simulink model "m2asm_2_rust"  (R2020b)
settings: Solver=FixedStepDiscrete  StartTime=0.0  StopTime=5  FixedStep=deltaT  RelTol=1e-3
values from neighbouring files (symbols this model uses):
  Cpi_d = c2d(st.asm.fpi,Ts,c2d_opts)    [load_m2asm_data.m]
  fc = 2    [load_m2asm_data.m]
  flag_d = c2d(flag,Ts,c2d_opts)    [load_m2asm_data.m]
  Hpd_d = c2d(st.asm.fpd,Ts,c2d_opts)    [load_m2asm_data.m]
  k2p_stiff = k2p_stiff0    (= 122000000)    [load_m2asm_data.m]
  Km2pS1_dec = Km2p_dec(1:6,1:6)    [load_m2asm_data.m]
  m2p_Cfb_d = c2d(tf(fbH), Ts, 'foh')    [load_m2asm_data.m]
  st = getcontrol_asm()    [load_m2asm_data.m]
  to_diff_m2p_F = kron(eye(6),[1;-1])    [load_m2asm_data.m]
settings Model: SimulationMode=accelerator  Creator=RRomano  LastModifiedBy=rromano
settings DataIOCC: SaveOutput=off  SignalLogging=off  DSMLogging=off  SaveTime=off  ReturnWorkspaceOutputs=off
settings OptimizationCC: StrengthReduction=on  PassReuseOutputArgsAs=Individual arguments  EfficientMapNaN2IntZero=off  SimCompilerOptimization=on  AccelVerboseBuild=on  OptimizeBlockOrder=speed  OptimizationPriority=Speed  OptimizationCustomize=off  MultiThreadedLoops=on  EfficientTunableParamExpr=on
settings DebuggingCC: InheritedTsInSrcMsg=none  MultiTaskRateTransMsg=warning  ParameterTunabilityLossMsg=error  SFUnexpectedBacktrackingDiag=warning  SFNoUnconditionalDefaultTransitionDiag=warning  SFExecutionAtInitializationDiag=none  ArithmeticOperatorsInVariantConditions=warning
settings HardwareCC: ProdBitPerLong=64  ProdHWDeviceType=Intel->x86-64 (Linux 64)  TargetBitPerLong=64  TargetBitPerPointer=64  TargetBitPerSizeT=64  TargetBitPerPtrDiffT=64  TargetLongLongMode=on  TargetIntDivRoundTo=Zero  TargetEndianess=LittleEndian  TargetWordSize=64  TargetHWDeviceType=MATLAB Host  ProdEqTarget=off
settings SFSimCC: SimUseLocalCustomCode=off  MATLABDynamicMemAlloc=off  CustomCodeUndefinedFunction=UseInterfaceOnly
settings RTWCC: Description=Embedded Coder  SystemTargetFile=ert.tlc  GenCodeOnly=on  TemplateMakefile=ert_default_tmf  GenerateReport=on  BuildConfiguration=Faster Runs  IncludeHyperlinkInReport=on  GenerateTraceInfo=on  GenerateTraceReport=on  GenerateTraceReportSl=on  GenerateTraceReportSf=on  GenerateTraceReportEml=on
settings CodeAppCC: ForceParamTrailComments=on  IgnoreCustomStorageClasses=off  MaxIdLength=128  OperatorAnnotations=on  SimulinkDataObjDesc=on  SFDataObjDesc=on  InsertBlockDesc=on  MATLABSourceComments=on
settings ERTTargetCC: GenerateSampleERTMain=on  SuppressErrorStatus=on  CodeInterfacePackaging=Reusable function  RootIOFormat=Structure reference  ERTCustomFileTemplate=example_file_process.tlc
settings ConfigComp: CovMetricSettings=dw  CovSaveCumulativeToWorkspaceVar=on  CovSaveSingleToWorkspaceVar=on  CovExternalEMLEnable=off

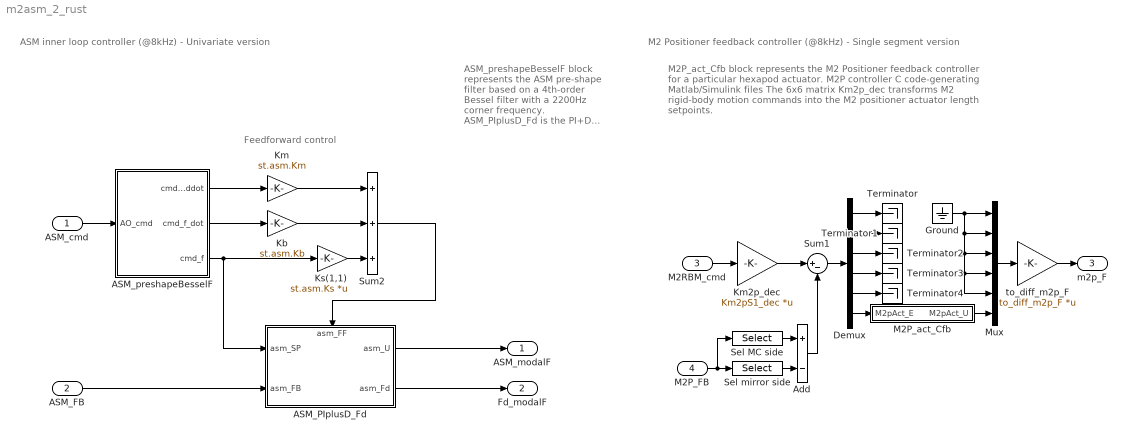
== system m2asm_2_rust ==
  note: Feedforward control
  note: ASM_preshapeBesselF block represents the ASM pre-shape filter based on a 4th-order Bessel filter with a 2200Hz corner frequency.
      | ASM_PIplusD_Fd is the PI+D feedback controller. The block also provides the fluid damping contribution as output asm_Fd .
      | In the modal control approach, Ks is the inverse of the modal stiffness matrix, a square matrix of dimension n_m. Therefore, in that case, Ks(1,1) is just a placeholder.
  note: ASM inner loop controller (@8kHz) - Univariate version
  note: M2 Positioner feedback controller (@8kHz) - Single segment version
  note: M2P_act_Cfb block represents the M2 Positioner feedback controller for a particular hexapod actuator.
      | M2P controller C code-generating Matlab/Simulink files
      | The 6x6 matrix Km2p_dec transforms M2 rigid-body motion commands into the M2 positioner actuator length setpoints.
  ASM_cmd : Inport  Interpolate=off
  ASM_FB : Inport  Port=2
  M2RBM_cmd : Inport  Port=3  Interpolate=off
  M2P_FB : Inport  Port=4
  ASM_PIplusD_Fd : Subsystem
      settings: PortSchema="{\"entries\":[{\"content\":{\"sides\":[{\"content\":{\"connectorIds\":[\"In1\",\"In2\"]},\"type\":\"ConnectorPlacement.EquallySpacedRectSide\",\"uuid\":\"706a4ecf-f719-44ad-a306-9c11e57cb316\"},{\"content\":{\"connectorIds\":[\"Out1\",\"Out2\"],\"side\":\"RIGHT\"},\"type\":\"ConnectorPlacement.EquallySpacedRectSide\",\"uuid\":\"04f8501d-a7a5-4c7b-93f1-e2b34d7c8dac\"},{\"content\":{\"connectorIds\":[\"In3\"],\"side\":\"TOP\"},\"type\":\"ConnectorPlacement.EquallySpacedRectSide\",\"uuid\":\"7dc3ff34-2b4e-4efd-8743-462d0862980d\"},{\"content\":{\"connectorIds\":[],\"side\":\"HIDDEN\"},\"type\":\"ConnectorPlacement.EquallySpacedRectSide\",\"uuid\":\"673e63a6-b266-47a9-b9c4-9219546d9f5b\"}]},\"type\":\"ConnectorPlacement.EquallySpacedConnector\",\"uuid\":\"903795e5-c455-47ea-8916-0bf0c79c1da5\"}],\"packageUris\":[\"http://schema.mathworks.com/mf0/Connector/R2020b\"],\"version\":\"1.0\"}"
  ASM_preshapeBesselF : Subsystem
  Add : Sum  Inputs=+-
  Demux : Demux  Outputs=6
  Ground : Ground
  Kb : Gain  Gain=st.asm.Kb
  Km : Gain  Gain=st.asm.Km
  Km2p_dec : Gain  Gain=Km2pS1_dec  Multiplication=Matrix(K*u) (u vector)
  Ks(1,1) : Gain  Gain=st.asm.Ks  Multiplication=Matrix(K*u)
  M2P_act_Cfb : Subsystem
  Mux : Mux  Inputs=6
  Sel MC side : Selector  InputPortWidth=12  IndexOptions=Index vector (dialog)  Indices=[1:2:12]  OutputSizes=1
  Sel mirror side : Selector  InputPortWidth=12  IndexOptions=Index vector (dialog)  Indices=[2:2:12]  OutputSizes=1
  Sum1 : Sum  Inputs=|+-
  Sum2 : Sum  Inputs=+++
  Terminator{,1..4} (5 alike) : Terminator
  to_diff_m2p_F : Gain  Gain=to_diff_m2p_F  Multiplication=Matrix(K*u)
  ASM_modalF : Outport  VectorParamsAs1DForOutWhenUnconnected=off
  Fd_modalF : Outport  Port=2  VectorParamsAs1DForOutWhenUnconnected=off
  m2p_F : Outport  Port=3  VectorParamsAs1DForOutWhenUnconnected=off
  wires:
  ASM_PIplusD_Fd/1(asm_U) -> ASM_modalF/1
  Sum2/1 -> ASM_PIplusD_Fd/3(asm_FF)
  Km/1 -> Sum2/1
  Kb/1 -> Sum2/2
  Ks(1,1)/1 -> Sum2/3
  ASM_cmd/1 -> ASM_preshapeBesselF/1(AO_cmd)
  ASM_preshapeBesselF/3(cmd_f) -> ASM_PIplusD_Fd/1(asm_SP), Ks(1,1)/1
  ASM_preshapeBesselF/2(cmd_f_dot) -> Kb/1
  ASM_FB/1 -> ASM_PIplusD_Fd/2(asm_FB)
  ASM_PIplusD_Fd/2(asm_Fd) -> Fd_modalF/1
  ASM_preshapeBesselF/1(cmd_f_ddot) -> Km/1
  M2RBM_cmd/1 -> Km2p_dec/1
  Km2p_dec/1 -> Sum1/1
  Add/1 -> Sum1/2
  Sum1/1 -> Demux/1
  Mux/1 -> to_diff_m2p_F/1
  to_diff_m2p_F/1 -> m2p_F/1
  Sel MC side/1 -> Add/1
  Sel mirror side/1 -> Add/2
  M2P_FB/1 -> Sel MC side/1, Sel mirror side/1
  Demux/1 -> Terminator/1
  Demux/2 -> Terminator1/1
  Demux/3 -> Terminator2/1
  Demux/4 -> Terminator3/1
  Demux/5 -> Terminator4/1
  Ground/1 -> Mux/5, Mux/4, Mux/3, Mux/2, Mux/1
  Demux/6 -> M2P_act_Cfb/1(M2pAct_E)
  M2P_act_Cfb/1(M2pAct_U) -> Mux/6

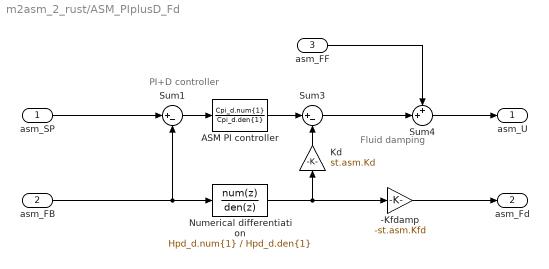
== system m2asm_2_rust/ASM_PIplusD_Fd ==
  note: PI+D controller
  note: Fluid damping
  asm_SP : Inport
  asm_FB : Inport  Port=2
  asm_FF : Inport  Port=3
  -Kfdamp : Gain  Gain=-st.asm.Kfd
  ASM PI controller : DiscreteTransferFcn  Numerator=Cpi_d.num{1}  Denominator=Cpi_d.den{1}  SampleTime=Cpi_d.Ts
  Kd : Gain  Gain=st.asm.Kd
  Numerical differentiation : DiscreteTransferFcn  Numerator=Hpd_d.num{1}  Denominator=Hpd_d.den{1}  SampleTime=Hpd_d.Ts
  Sum1 : Sum  Inputs=|+-
  Sum3 : Sum  Inputs=|+-
  Sum4 : Sum  Inputs=++|
  asm_U : Outport
  asm_Fd : Outport  Port=2
  wires:
  Kd/1 -> Sum3/2
  ASM PI controller/1 -> Sum3/1
  asm_SP/1 -> Sum1/1
  Numerical differentiation/1 -> -Kfdamp/1, Kd/1
  asm_FB/1 -> Numerical differentiation/1, Sum1/2
  Sum1/1 -> ASM PI controller/1
  -Kfdamp/1 -> asm_Fd/1
  Sum3/1 -> Sum4/2
  asm_FF/1 -> Sum4/1
  Sum4/1 -> asm_U/1

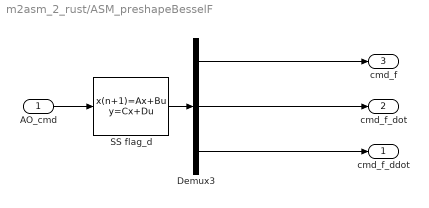
== system m2asm_2_rust/ASM_preshapeBesselF ==
  AO_cmd : Inport
  Demux3 : Demux  Outputs=3
  SS flag_d : DiscreteStateSpace  A=flag_d.A  B=flag_d.B  C=flag_d.C  D=flag_d.D  SampleTime=flag_d.Ts
  cmd_f_ddot : Outport
  cmd_f_dot : Outport  Port=2
  cmd_f : Outport  Port=3
  wires:
  Demux3/1 -> cmd_f/1
  Demux3/3 -> cmd_f_ddot/1
  Demux3/2 -> cmd_f_dot/1
  AO_cmd/1 -> SS flag_d/1
  SS flag_d/1 -> Demux3/1

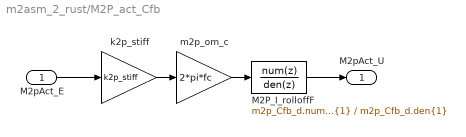
== system m2asm_2_rust/M2P_act_Cfb ==
  M2pAct_E : Inport
  M2P_I_rolloffF : DiscreteTransferFcn  Numerator=m2p_Cfb_d.num{1}  Denominator=m2p_Cfb_d.den{1}  SampleTime=m2p_Cfb_d.Ts
  k2p_stiff : Gain  Gain=k2p_stiff
  m2p_om_c : Gain  Gain=2*pi*fc
  M2pAct_U : Outport
  wires:
  M2P_I_rolloffF/1 -> M2pAct_U/1
  M2pAct_E/1 -> k2p_stiff/1
  k2p_stiff/1 -> m2p_om_c/1
  m2p_om_c/1 -> M2P_I_rolloffF/1
